simulink model "VOO"  (R2020a)
settings: Solver=FixedStepAuto  StartTime=0.0  StopTime=inf  FixedStep=0.001  RelTol=1e-3  EnableMultiTasking=on
undefined symbols (not defined in the file): D10, D11, D12, D2, D4, D5, D7, D8, D9, PTA0, PTA2, PTB23, PTB9, PTC3, PTC4, PTD0, PTD2, PTD3
libraries: frdmk64flib x9
settings Model: ExtModeTrigDuration=5  Creator=12268  LastModifiedBy=12268
settings OptimizationCC: EnhancedBackFolding=on  PassReuseOutputArgsAs=Individual arguments  ZeroExternalMemoryAtStartup=off  ZeroInternalMemoryAtStartup=off  MaxStackSize=64  OptimizeBlockOrder=speed  DifferentSizesBufferReuse=on  OptimizationCustomize=off  EfficientTunableParamExpr=on
settings DebuggingCC: ParameterTunabilityLossMsg=error
settings HardwareCC: ProdBitPerPointer=32  ProdBitPerSizeT=32  ProdBitPerPtrDiffT=32  ProdLargestAtomicInteger=Long  ProdLargestAtomicFloat=Double  ProdWordSize=32  ProdHWDeviceType=ARM Compatible->ARM Cortex
settings SFSimCC: MATLABDynamicMemAlloc=off
settings RTWCC: SystemTargetFile=ert.tlc  HardwareBoard=NXP FRDM-K64F  TemplateMakefile=ert_default_tmf  Toolchain=GNU Tools for ARM Embedded Processors
settings CodeAppCC: ForceParamTrailComments=on  IgnoreCustomStorageClasses=off  OperatorAnnotations=on  SimulinkDataObjDesc=on  SFDataObjDesc=on  InsertBlockDesc=on

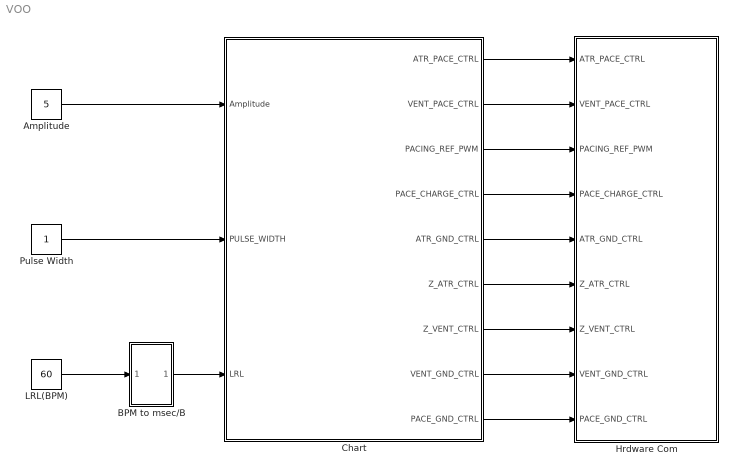
== system VOO ==
  Amplitude : Constant  Value=5  OutDataTypeStr=double
  "BPM to msec/B " : Subsystem
  Chart : Stateflow chart  TreatAsAtomicUnit=on
  Hrdware Com : Subsystem
  LRL(BPM) : Constant  Value=60  OutDataTypeStr=double
  Pulse Width : Constant  OutDataTypeStr=uint16
  wires:
  Chart/1(ATR_PACE_CTRL) -> Hrdware Com/1(ATR_PACE_CTRL)
  Amplitude/1 -> Chart/1(Amplitude)
  Chart/9(PACE_GND_CTRL) -> Hrdware Com/9(PACE_GND_CTRL)
  Chart/3(PACING_REF_PWM) -> Hrdware Com/3(PACING_REF_PWM)
  Chart/2(VENT_PACE_CTRL) -> Hrdware Com/2(VENT_PACE_CTRL)
  Chart/4(PACE_CHARGE_CTRL) -> Hrdware Com/4(PACE_CHARGE_CTRL)
  Chart/5(ATR_GND_CTRL) -> Hrdware Com/5(ATR_GND_CTRL)
  Chart/6(Z_ATR_CTRL) -> Hrdware Com/6("Z_ATR_CTRL ")
  Chart/7(Z_VENT_CTRL) -> Hrdware Com/7("Z_VENT_CTRL ")
  Chart/8(VENT_GND_CTRL) -> Hrdware Com/8(VENT_GND_CTRL)
  Pulse Width/1 -> Chart/2(PULSE_WIDTH)
  "BPM to msec/B "/1(Out1) -> Chart/3(LRL)
  LRL(BPM)/1 -> "BPM to msec/B "/1(In1)

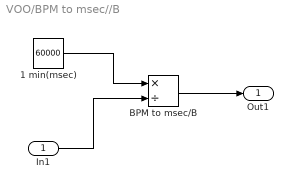
== system VOO/BPM to msec//B  ==
  In1 : Inport
  1 min(msec) : Constant  Value=60000  OutDataTypeStr=double
  "BPM to msec/B " : Product  Inputs=*/  OutDataTypeStr=uint16  RndMeth=Nearest
  Out1 : Outport
  wires:
  1 min(msec)/1 -> "BPM to msec/B "/1
  "BPM to msec/B "/1 -> Out1/1
  In1/1 -> "BPM to msec/B "/2

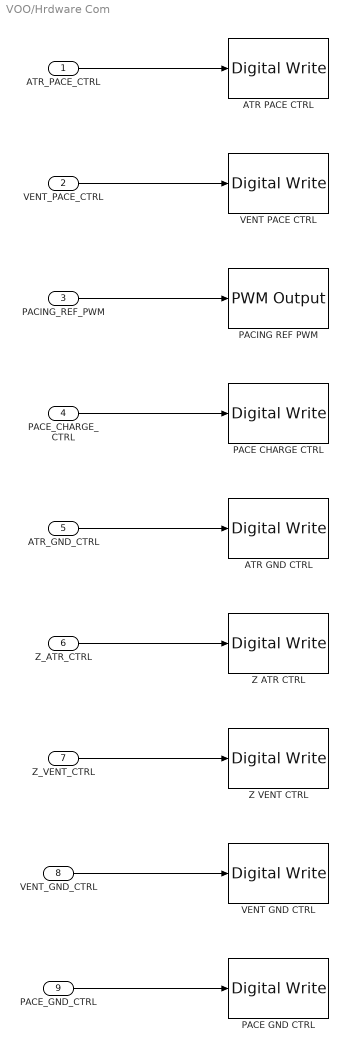
== system VOO/Hrdware Com ==
  ATR_PACE_CTRL : Inport
  VENT_PACE_CTRL : Inport  Port=2
  PACING_REF_PWM : Inport  Port=3
  PACE_CHARGE_CTRL : Inport  Port=4
  ATR_GND_CTRL : Inport  Port=5
  "Z_ATR_CTRL " : Inport  Port=6
  "Z_VENT_CTRL " : Inport  Port=7
  VENT_GND_CTRL : Inport  Port=8
  PACE_GND_CTRL : Inport  Port=9
  "ATR GND CTRL " : frdmk64flib/Digital Write  Whichpin=PTD2 (D11)
  ATR PACE CTRL : frdmk64flib/Digital Write  Whichpin=PTA0 (D8)
  PACE CHARGE CTRL : frdmk64flib/Digital Write  Whichpin=PTB9 (D2)
  PACE GND CTRL : frdmk64flib/Digital Write  Whichpin=PTD0 (D10)
  PACING REF PWM : frdmk64flib/PWM Output  Whichpin=PTA2 (D5)  InitialFrequency=2000  InitialDutyCycle=0
  VENT GND CTRL : frdmk64flib/Digital Write  Whichpin=PTD3 (D12)
  VENT PACE CTRL : frdmk64flib/Digital Write  Whichpin=PTC4 (D9)
  "Z ATR CTRL " : frdmk64flib/Digital Write  Whichpin=PTB23 (D4)
  "Z VENT CTRL " : frdmk64flib/Digital Write  Whichpin=PTC3 (D7)
  wires:
  ATR_PACE_CTRL/1 -> ATR PACE CTRL/1
  VENT_PACE_CTRL/1 -> VENT PACE CTRL/1
  PACING_REF_PWM/1 -> PACING REF PWM/1
  PACE_CHARGE_CTRL/1 -> PACE CHARGE CTRL/1
  ATR_GND_CTRL/1 -> "ATR GND CTRL "/1
  "Z_ATR_CTRL "/1 -> "Z ATR CTRL "/1
  "Z_VENT_CTRL "/1 -> "Z VENT CTRL "/1
  VENT_GND_CTRL/1 -> VENT GND CTRL/1
  PACE_GND_CTRL/1 -> PACE GND CTRL/1

== stateflow chart VOO/Chart ==
  state Charging_and_Discharging
    entry:
    PACE_GND_CTRL=true;
    ATR_PACE_CTRL=false;
    VENT_PACE_CTRL=false;
    PACING_REF_PWM=uint8(Amplitude*20);
    PACE_CHARGE_CTRL=true;
    Z_ATR_CTRL=false;
    Z_VENT_CTRL=false;
    ATR_GND_CTRL=false;
    VENT_GND_CTRL=true;
  state V_Pacing
    entry:
    PACE_CHARGE_CTRL=false;
    PACE_GND_CTRL=true;
    ATR_GND_CTRL=false;
    Z_ATR_CTRL=false;
    Z_VENT_CTRL=false;
    VENT_GND_CTRL=false;
    ATR_PACE_CTRL=false;
    VENT_PACE_CTRL=true;
  (default) -> Charging_and_Discharging
  Charging_and_Discharging -> V_Pacing : after(LRL-PULSE_WIDTH, msec)
  V_Pacing -> Charging_and_Discharging : after(PULSE_WIDTH, msec)
  data: ATR_PACE_CTRL output boolean; VENT_PACE_CTRL output boolean; PACING_REF_PWM output uint8; Amplitude input double; PACE_CHARGE_CTRL output boolean; ATR_GND_CTRL output boolean; Z_ATR_CTRL output boolean; Z_VENT_CTRL output boolean; VENT_GND_CTRL output boolean; PACE_GND_CTRL output boolean; PULSE_WIDTH input uint16; LRL input uint16
